simulink model "diagrama_bloques"  (R2026a)
settings: Solver=VariableStepAuto
settings Model: Creator=pablo  LastModifiedBy=pablo

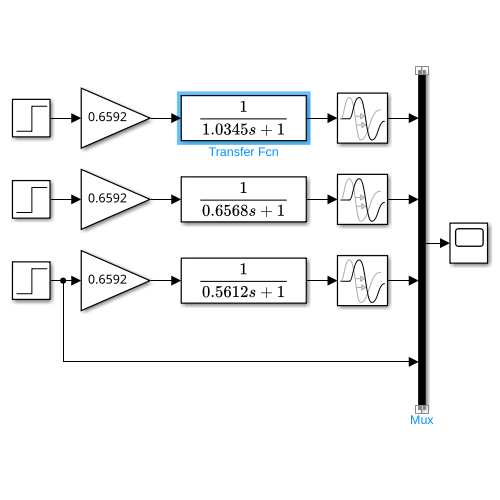
[thumbnail: Simulink's stored preview of the top-level diagram]
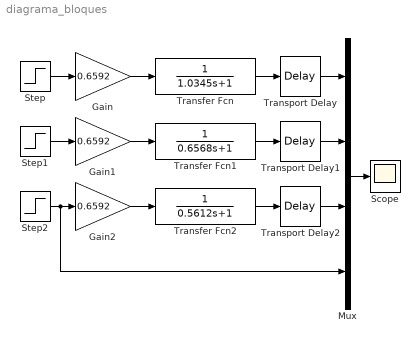
== system diagrama_bloques ==
  Gain : Gain  Gain=0.6592
  Gain1 : Gain  Gain=0.6592
  Gain2 : Gain  Gain=0.6592
  Mux : Mux
  Scope : Scope
      settings: ActiveDisplayYMinimum=-0.12499999999999997  ActiveDisplayYMaximum=1.125
  Step : Step  SampleTime=0
  Step1 : Step  SampleTime=0
  Step2 : Step  SampleTime=0
  Transfer Fcn : TransferFcn  Denominator=[1.0345 1]
  Transfer Fcn1 : TransferFcn  Denominator=[0.6568 1]
  Transfer Fcn2 : TransferFcn  Denominator=[0.5612 1]
  Transport Delay : TransportDelay  DelayTime=0.059
  Transport Delay1 : TransportDelay  DelayTime=0.059
  Transport Delay2 : TransportDelay  DelayTime=0.1545
  wires:
  Step/1 -> Gain/1
  Gain/1 -> Transfer Fcn/1
  Transfer Fcn/1 -> Transport Delay/1
  Transport Delay/1 -> Mux/1
  Step1/1 -> Gain1/1
  Gain1/1 -> Transfer Fcn1/1
  Transfer Fcn1/1 -> Transport Delay1/1
  Gain2/1 -> Transfer Fcn2/1
  Transfer Fcn2/1 -> Transport Delay2/1
  Transport Delay1/1 -> Mux/2
  Transport Delay2/1 -> Mux/3
  Step2/1 -> Mux/4, Gain2/1
  Mux/1 -> Scope/1
